simulink model "Ejercicio25_8_sim"  (R2023b)
settings: Solver=VariableStepAuto  StartTime=0.0  StopTime=inf  MaxStep=1e-3  RelTol=1e-3
values from neighbouring files (symbols this model uses):
  b = 1    [Ejercicio11_8.m]    (also in Ejercicio25_8.m)
  g = 9.806    [Ejercicio25_8.m]
  m = 1    [Ejercicio25_8.m]
libraries: simulink x3, slpidlib x1
settings Model: PacingRate=0.500000  Creator=tomas  LastModifiedBy=tomas

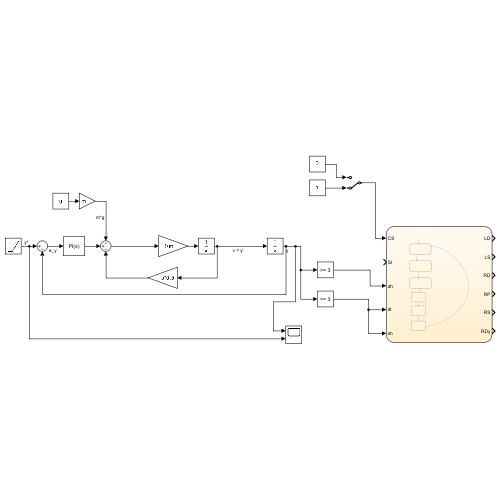
[thumbnail: Simulink's stored preview of the top-level diagram]
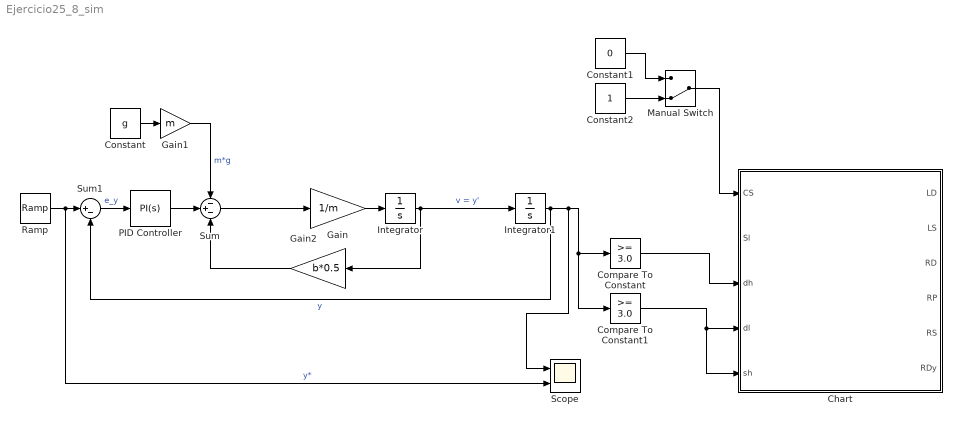
== system Ejercicio25_8_sim ==
  Chart : Stateflow chart  TreatAsAtomicUnit=on
      settings: PortSchema="{\"entries\":[{\"content\":{\"sides\":[{\"content\":{\"connectorIds\":[\"In4\",\"In5\",\"In1\",\"In2\",\"In3\"]},\"type\":\"ConnectorPlacement.EquallySpacedRectSide\",\"uuid\":\"6b7303d2-480e-44b0-b7c3-94d333f1b8b1\"},{\"content\":{\"connectorIds\":[\"Out1\",\"Out2\",\"Out3\",\"Out4\",\"Out5\",\"Out6\"],\"side\":\"RIGHT\"},\"type\":\"ConnectorPlacement.EquallySpacedRectSide\",\"uuid\":\"71ac8057-29c1-4d4e-8ea0-4bf40e98a52c\"},{\"content\":{\"side\":\"TOP\"},\"type\":\"ConnectorPlacement.EquallySpacedRectSide\",\"uuid\":\"f4b319d7-6502-4e16-864b-da40d118378a\"}]},\"type\":\"ConnectorPlacement.EquallySpacedConnector\",\"uuid\":\"83f91d81-97ec-4c41-80d5-92e73eb33486\"}],\"packageUris\":[\"http://schema.mathworks.com/mf0/Connector/R2020b\"],\"version\":\"1.0\"}"
  Compare To Constant : simulink/Logic and Bit Operations/Compare To Constant  relop=>=  const=3.0  OutDataTypeStr=boolean
  Compare To Constant1 : simulink/Logic and Bit Operations/Compare To Constant  relop=>=  const=3.0  OutDataTypeStr=boolean
  Constant : Constant  Value=g
  Constant1 : Constant  Value=0
  Constant2 : Constant
  Gain : Gain  Gain=1/m
  Gain1 : Gain  Gain=m
  Gain2 : Gain  Gain=b*0.5
  Integrator : Integrator
  Integrator1 : Integrator
  Manual Switch : ManualSwitch  CurrentSetting=0
  PID Controller : slpidlib/PID Controller  Controller=PI  Form=Parallel  TimeDomain=Continuous-time  UseExternalTs=off  SampleTime=-1  IntegratorMethod=Forward Euler  FilterMethod=Forward Euler  ControllerParametersSource=internal  P=1  I=0.5  UseKiTs=off  D=0  N=100  UseFilter=on  TunerSelectOption=Transfer Function Based (PID Tuner App)  InitialConditionSource=internal  InitialConditionForIntegrator=0  InitialConditionForFilter=0  DifferentiatorICPrevScaledInput=0  ExternalReset=none  TrackingMode=off  Kt=1  LimitOutput=off  SatLimitsSource=internal  UpperSaturationLimit=inf  LowerSaturationLimit=-inf  LinearizeAsGain=on  AntiWindupMode=none  Kb=1  LimitIntegrator=off  UpperIntegratorSaturationLimit=inf  LowerIntegratorSaturationLimit=-inf  POutMin=[]  POutMax=[]  IOutMin=[]  IOutMax=[]  DOutMin=[]  DOutMax=[]  NOutMin=[]  NOutMax=[]  SumOutMin=[]  SumOutMax=[]  SaturationOutMin=[]  SaturationOutMax=[]  PParamMin=[]  PParamMax=[]  IParamMin=[]  IParamMax=[]  DParamMin=[]  DParamMax=[]  NParamMin=[]  NParamMax=[]  KbParamMin=[]  KbParamMax=[]  KtParamMin=[]  KtParamMax=[]  KbOutMin=[]  KbOutMax=[]  KtOutMin=[]  KtOutMax=[]  IntegratorOutMin=[]  IntegratorOutMax=[]  FilterOutMin=[]  FilterOutMax=[]  SumI1OutMin=[]  SumI1OutMax=[]  SumI2OutMin=[]  SumI2OutMax=[]  SumI3OutMin=[]  SumI3OutMax=[]  SumI4OutMin=[]  SumI4OutMax=[]  SumDOutMin=[]  SumDOutMax=[]  DifferentiatorOutMin=[]  DifferentiatorOutMax=[]  FilterDiffOutCoefMin=[]  FilterDiffOutCoefMax=[]  ReciprocalOutMin=[]  ReciprocalOutMax=[]  SumDenOutMin=[]  SumDenOutMax=[]  SumNumOutMin=[]  SumNumOutMax=[]  DivideOutMin=[]  DivideOutMax=[]  UdiffTsProdOutMin=[]  UdiffTsProdOutMax=[]  NTsProdOutMin=[]  NTsProdOutMax=[]  UintegralTsProdOutMin=[]  UintegralTsProdOutMax=[]  UngainTsProdOutMin=[]  UngainTsProdOutMax=[]  ClampingZeroOutDataTypeStr=Inherit: Inherit via back propagation  ClampingZeroOutMin=[]  ClampingZeroOutMax=[]  FilterDenConstantOutDataTypeStr=Inherit: Inherit via back propagation  FilterDenConstantOutMin=[]  FilterDenConstantOutMax=[]  PCopyOutDataTypeStr=Inherit: Inherit via back propagation  PCopyOutMin=[]  PCopyOutMax=[]  NCopyOutDataTypeStr=Inherit: Inherit via back propagation  NCopyOutMin=[]  NCopyOutMax=[]  IntegratorContinuousStateAttributes=''  IntegratorStateMustResolveToSignalObject=off  IntegratorRTWStateStorageClass=Auto  FilterContinuousStateAttributes=''  FilterStateMustResolveToSignalObject=off  FilterRTWStateStorageClass=Auto  ParallelPVariant=InternalParameters  IdealPVariant=Disabled  IVariant=InternalParameters  DVariant=Disabled  IntegratorVariant=Continuous  SatVariant=Disabled  AWVariant=Passthrough  PCopyVariant=Disabled  TRVariant=Disabled  FdbkBlocksVariant=Forward  IdealPFdbkVariant=Disabled  SatFdbkVariant=Disabled  DerivativeFilterVariant=Disabled  NVariant=Disabled  NCopyVariant=Disabled_SignalSpec  FilterICVariant=Disabled  IntegratorICVariant=InternalICs  ExternalResetVariant=Disabled  TRSumVariant=Passthrough  SumFdbkVariant=Disabled  SumVariant=Sum_PI  TsampFilterVariant=InternalTs  TsampNgainVariant=Passthrough  TsampIntegralVariant=Disabled_SignalSpec  ExternalSaturationOutDataTypeStr=Inherit: Same as second input
  Ramp : simulink/Sources/Ramp  slope=1  start=0  InitialOutput=0
  Scope : Scope  NumInputPorts=2
  Sum : Sum  Inputs=-+-
  Sum1 : Sum  Inputs=|+-
  wires:
  Integrator/1 -> Integrator1/1, Gain2/1  "v = y'"
  Constant/1 -> Gain1/1
  Sum/1 -> Gain/1
  Gain2/1 -> Sum/3
  Ramp/1 -> Scope/2, Sum1/1  "y*"
  Gain/1 -> Integrator/1
  Gain1/1 -> Sum/1  "m*g"
  Integrator1/1 -> Sum1/2, Scope/1, Compare To Constant1/1, Compare To Constant/1  "y"
  Constant1/1 -> Manual Switch/1
  Constant2/1 -> Manual Switch/2
  Manual Switch/1 -> Chart/4(CS)
  Compare To Constant/1 -> Chart/1(dh)
  Compare To Constant1/1 -> Chart/3(sh), Chart/2(dl)
  Sum1/1 -> PID Controller/1  "e_y"
  PID Controller/1 -> Sum/2

== stateflow chart Ejercicio25_8_sim/Chart ==
  state Estado1_Reposo
    du: RDy = (sh && dh);
  state Estado2_BajarPunzon
    entry: LS = 1;
    exit:  LS = 0;
  state Estado3_SubirPunzon
    entry: RS = 1;
    exit:  RS = 0;
  state Estado4_BajarMatriz
    entry: LD = 1;
    exit:  LD = 0;
  state Estado5_RemoverPieza
    entry: RP = 1;
    exit:  RP = 0;
  state Estado6_SubirMatriz
    entry: RD = 1;
    exit:  RD = 0;
  (default) -> Estado1_Reposo
  Estado6_SubirMatriz -> Estado1_Reposo : [dh]
  Estado1_Reposo -> Estado2_BajarPunzon : [CS && sh && dh]
  Estado2_BajarPunzon -> Estado3_SubirPunzon : [Sl]
  Estado3_SubirPunzon -> Estado4_BajarMatriz : [sh]
  Estado4_BajarMatriz -> Estado5_RemoverPieza : [dl]
  Estado5_RemoverPieza -> Estado6_SubirMatriz : after(5, sec)
  data: dh input; dl input; sh input; LD output; LS output; RD output; RP output; RS output; RDy output; CS input; Sl input
